simulink model "iso_calc_temp_ver4"  (R2020a)
settings: Solver=VariableStepAuto  StartTime=0.0  StopTime=inf  RelTol=1e-6
undefined symbols (not defined in the file): C, t_current, Tr, Ts, Vs, Zd, Zr
settings Model: Creator=laiy  LastModifiedBy=laiy

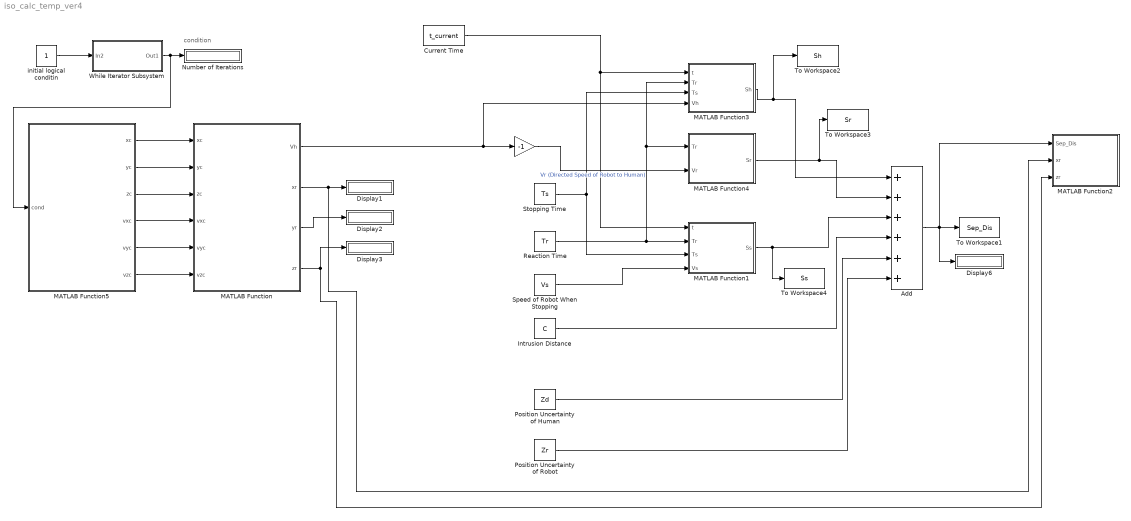
== system iso_calc_temp_ver4 ==
  note: condition
  " " : Gain  Gain=-1
  Add : Sum  Inputs=++++++
  Current Time : Constant  Value=t_current
  Display{1..3,6} (4 alike) : Display
  Intrusion Distance : Constant  Value=C
  MATLAB Function : MATLAB Function  TreatAsAtomicUnit=on
  MATLAB Function1 : MATLAB Function  TreatAsAtomicUnit=on
  MATLAB Function2 : MATLAB Function  TreatAsAtomicUnit=on
  MATLAB Function3 : MATLAB Function  TreatAsAtomicUnit=on
  MATLAB Function4 : MATLAB Function  TreatAsAtomicUnit=on
  MATLAB Function5 : MATLAB Function  TreatAsAtomicUnit=on
  Number of Iterations : Display
  Position Uncertainty of Human : Constant  Value=Zd
  Position Uncertainty of Robot : Constant  Value=Zr
  Reaction Time : Constant  Value=Tr
  Speed of Robot When Stopping : Constant  Value=Vs
  Stopping Time : Constant  Value=Ts
  To Workspace1 : ToWorkspace  VariableName=Sep_Dis  SampleTime=-1
  To Workspace2 : ToWorkspace  VariableName=Sh  SampleTime=-1
  To Workspace3 : ToWorkspace  VariableName=Sr  SampleTime=-1
  To Workspace4 : ToWorkspace  VariableName=Ss  SampleTime=-1
  While Iterator Subsystem : Subsystem  TreatAsAtomicUnit=on
  initial logical conditin : Constant
  wires:
  MATLAB Function1/1(Ss) -> To Workspace4/1, Add/3
  MATLAB Function3/1(Sh) -> To Workspace2/1, Add/1
  MATLAB Function4/1(Sr) -> To Workspace3/1, Add/2
  Intrusion Distance/1 -> Add/4
  Position Uncertainty of Human/1 -> Add/5
  Position Uncertainty of Robot/1 -> Add/6
  Reaction Time/1 -> MATLAB Function1/2(Tr), MATLAB Function4/1(Tr), MATLAB Function3/2(Tr)
  Stopping Time/1 -> MATLAB Function3/3(Ts), MATLAB Function1/3(Ts)
  " "/1 -> MATLAB Function4/2(Vr)  "Vr (Directed Speed of Robot to Human)"
  Current Time/1 -> MATLAB Function1/1(t), MATLAB Function3/1(t)
  Speed of Robot When Stopping/1 -> MATLAB Function1/4(Vs)
  Add/1 -> MATLAB Function2/1(Sep_Dis), Display6/1, To Workspace1/1
  MATLAB Function/1(Vh) -> MATLAB Function3/4(Vh), " "/1
  MATLAB Function/2(xr) -> MATLAB Function2/2(xr), Display1/1
  MATLAB Function/3(yr) -> Display2/1
  MATLAB Function5/1(xc) -> MATLAB Function/1(xc)
  MATLAB Function5/2(yc) -> MATLAB Function/2(yc)
  MATLAB Function5/3(zc) -> MATLAB Function/3(zc)
  MATLAB Function5/4(vxc) -> MATLAB Function/4(vxc)
  MATLAB Function5/5(vyc) -> MATLAB Function/5(vyc)
  MATLAB Function5/6(vzc) -> MATLAB Function/6(vzc)
  MATLAB Function/4(zr) -> MATLAB Function2/3(zr), Display3/1
  While Iterator Subsystem/1(Out1) -> MATLAB Function5/1(cond), Number of Iterations/1
  initial logical conditin/1 -> While Iterator Subsystem/1(In2)

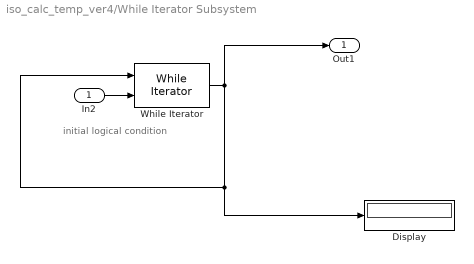
== system iso_calc_temp_ver4/While Iterator Subsystem ==
  note: initial logical
      | condition
  In2 : Inport
  Display : Display
  While Iterator : WhileIterator  MaxIters=1  ResetStates=reset  ShowIterationPort=on
  Out1 : Outport  VectorParamsAs1DForOutWhenUnconnected=off
  wires:
  In2/1 -> While Iterator/2
  While Iterator/1 -> Out1/1, Display/1, While Iterator/1

== matlab function iso_calc_temp_ver4/MATLAB Function4 ==
  data: Tr input; Vr input; Sr output
function Sr = fcn(Tr, Vr)

% separation distance due to robot motion
% Vr is assumed to reduces the separation distance the most

Sr = Tr * Vr;

== matlab function iso_calc_temp_ver4/MATLAB Function3 ==
  data: t input; Sh output; Tr input; Ts input; Vh input
function Sh = fcn(t, Tr, Ts, Vh)

% separation distance due to operator's change in location

%% Integral
% t_int = t:0.001:t+Tr+Ts;
% v = zeros(length(t_int),1) + Vh;
% 
% Sh = trapz(t_int,v);

%% Assuming Constant
Sh = (t+Tr+Ts) * Vh;

== matlab function iso_calc_temp_ver4/MATLAB Function1 ==
  data: t input; Tr input; Ss output; Ts input; Vs input
function Ss = fcn(t, Tr, Ts, Vs)

% separation distance due to robot stopping

%% Integral 
% t_int = t+Tr:0.001:t+Tr+Ts;
% v = zeros(length(t_int),1) + Vs;
% 
% Ss = trapz(t_int,v);

%% Assuming Constant
Ss = (t+Tr+Ts)*Vs;

== matlab function iso_calc_temp_ver4/MATLAB Function2 ==
  data: Sep_Dis input; xr input; zr input
function display(Sep_Dis, xr,zr)

% fprintf(1, 'Separation Distance: %f\n', Sep_Dis(1,1));

fileID = fopen('output.txt','w');
fprintf(fileID,'%f\n',Sep_Dis);
fclose(fileID);


% f = figure(1);
% title('Separation Distance');
% plot(xr*5,zr*5,'o','MarkerSize', 3, 'MarkerFaceColor', 'black');
% hold on;
% plot(0,0,'o','MarkerSize',1, 'LineWidth', 3, 'Color', 'Red','MarkerSize', int8(abs(Sep_Dis)*100));
% hold off;
% xlim([-5,5]);
% ylim([-5,5]);

if sqrt(xr^2 + zr^2) <= Sep_Dis
%     fprintf(1,'DANGER');
end

== matlab function iso_calc_temp_ver4/MATLAB Function ==
  data: xc input; Vh output; yc input; zc input; vxc input; vyc input; vzc input; xr output; yr output; zr output
function [Vh,xr,yr,zr] = find_Vh(xc,yc,zc,vxc,vyc,vzc)

[xr,yr,zr,vxr,vyr,vzr] = trans_cam_rob(xc,yc,zc,vxc,vyc,vzc);

Vh = sqrt(vxr^2 + vzr^2);

== matlab function iso_calc_temp_ver4/MATLAB Function5 ==
  data: xc output; yc output; zc output; vxc output; vyc output; vzc output; cond input
function [xc,yc,zc,vxc,vyc,vzc] = loopData(cond)

% rng shuffle
r = rand(1,6);
fprintf(1,'First Random: %f\n', r(1));

xc = 0;
yc = 0;
zc = 0;
vxc = 0;
vyc = 0;
vzc = 0;

if (cond)
    %TODO: replace below code with your data callback func
    xc = r(1);
    yc = r(2);
    zc = r(3);
    vxc = r(4);
    vyc = r(5);
    vzc = r(6);
end
